simulink model "battery_model_test1"  (R2015a)
settings: Solver=ode45  StartTime=0.0  StopTime=10.0  RelTol=1e-3
undefined symbols (not defined in the file or in its folder): Ion, Lithium
libraries: fl_lib x3, nesl_utility x2, electricdrivelib x1, powerlib x1
settings Model: Creator=satya  LastModifiedBy=satya

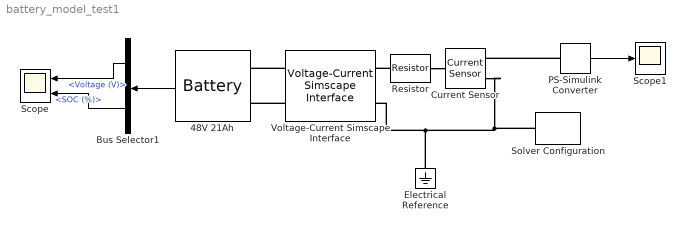
== system battery_model_test1 ==
  48V 21Ah : electricdrivelib/Extra Sources/Battery  BatType=Lithium-Ion  ShowDetailedParameters=off  NomV=48  NomQ=21  SOC=100  PresetModel=on  MaxQ=21  FullV=55.8714  Dis_rate=9.1304  R=0.022857  Normal_OP=18.9913  expZone="[51.8585      1.03174]"  current=[6.5 20 32.5]  Units=Time  Batt_Tr=30
  Bus Selector1 : BusSelector  OutputSignals=Voltage (V),SOC (%)
  Current Sensor : fl_lib/Electrical/Electrical Sensors/Current Sensor
  Electrical Reference : fl_lib/Electrical/Electrical Elements/Electrical Reference
  PS-Simulink Converter : nesl_utility/PS-Simulink Converter  PhysicalDomain=network_engine_domain  SubClassName=ps_output  LeftPortType=input  RightPortType=output  PseudoPeriodic=off  Frequencies=[]  Unit=1  AffineConversion=off
  Resistor : fl_lib/Electrical/Electrical Elements/Resistor  R=10 kOhm  i_specify=off  i_priority=High  i=0 A  v_specify=off  v_priority=High  v=0 V
  Scope : Scope  NumInputPorts=2
      settings: YMin=-5~-5  YMax=5~5
  Scope1 : Scope
  Solver Configuration : nesl_utility/Solver Configuration  PhysicalDomain=network_engine_domain  SubClassName=solver  LeftPortType=input  RightPortType=generic  Accelerate=off  Tones=[]  Harmonics=[]  SimulateNoise=off  Profile=off  UseLocalSampling=off  EnableSwitchedLinearOptims=on  FrequencyDomain=off  UseCCode=off  RelTol=0.001  AbsTol=1e-06  MinStep=1e-09  ToWorkspace=off  RevertToSquareIcSolve=off  NumHomotopyIterations=100  DoDC=off  ResidualTolerance=1e-09  UseLocalSolver=off  LocalSolverChoice=NE_BACKWARD_EULER_ADVANCER  LocalSolverSampleTime=0.001  DoFixedCost=off  MaxNonlinIter=3  MaxModeIter=2  LinearAlgebra=Sparse  DelaysMemoryBudget=1024  AutomaticFiltering=on  FilteringTimeConstant=0.001
  Voltage-Current Simscape Interface : powerlib/Interface Elements/Voltage-Current Simscape Interface  DFT=off  Fmode=Low pass filter (continuous)  T=1e-6  Ts=50e-6  i0=0  v0=0  Sd=SimPowerSystems side  Measurements=off
  wires:
  48V 21Ah/1 -> Bus Selector1/1
  PS-Simulink Converter/1 -> Scope1/1
  Bus Selector1/1 -> Scope/1  "<Voltage (V)>"
  Bus Selector1/2 -> Scope/2  "<SOC (%)>"
  connections:
  Voltage-Current Simscape Interface/LConn1 -- 48V 21Ah/LConn1
  Voltage-Current Simscape Interface/LConn2 -- 48V 21Ah/LConn2
  Current Sensor/RConn2 -- Solver Configuration/RConn1 -- Electrical Reference/LConn1 -- Voltage-Current Simscape Interface/RConn2
  PS-Simulink Converter/LConn1 -- Current Sensor/RConn1
  Resistor/LConn1 -- Voltage-Current Simscape Interface/RConn1
  Resistor/RConn1 -- Current Sensor/LConn1
